simulink model "Main"  (R2020b)
settings: Solver=FixedStepAuto  StartTime=0.0  StopTime=60  FixedStep=0.01  RelTol=1e-3
settings Model: Creator=kaebi  LastModifiedBy=kaebi
settings OptimizationCC: DefaultParameterBehavior=Inlined  LocalBlockOutputs=off
settings RTWCC: Description=TwinCAT GRT Target  SystemTargetFile=TwinCatGrt.tlc  GenCodeOnly=on  TemplateMakefile=tcgrt_msbuild.tmf  TargetLang=C++
settings STFCustomTargetCC: TargetLangStandard=C++03 (ISO)  ConcurrentExecutionCompliant=off  CombineOutputUpdateFcns=on  CodeInterfacePackaging=Reusable function  GRTInterface=off  GenerateAllocFcn=on  SystemTargetFile=TwinCatGrt.tlc
settings GRTTargetCC: TargetLangStandard=C++03 (ISO)  ParMdlRefBuildCompliant=off  CompOptLevelCompliant=off  ConcurrentExecutionCompliant=off  MatFileLogging=off  CodeInterfacePackaging=Reusable function  GenerateAllocFcn=on  UseToolchainInfoCompliant=off  ExtModeMexFile=TcExtModeClient

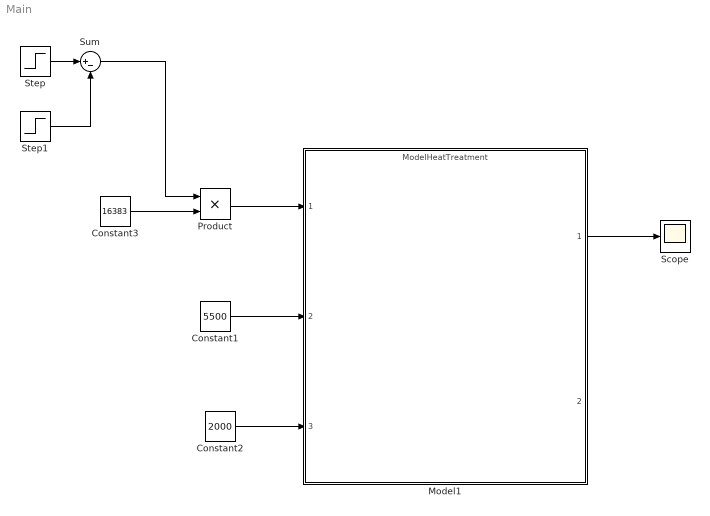
== system Main ==
  Constant1 : Constant  Value=5500  OutDataTypeStr=uint16
  Constant2 : Constant  Value=2000  OutDataTypeStr=uint16
  Constant3 : Constant  Value=16383  OutDataTypeStr=uint16
  Model1 : ModelReference  ModelNameDialog=ModelHeatTreatment.slx  SimulationMode=Normal  ModelReferenceVersion=1.35
  Product : Product  OutDataTypeStr=uint16
  Scope : Scope
  Step : Step  SampleTime=0
  Step1 : Step  Time=30  SampleTime=0
  Sum : Sum  Inputs=|+-
  wires:
  Model1/1 -> Scope/1
  Step/1 -> Sum/1
  Step1/1 -> Sum/2
  Product/1 -> Model1/1
  Constant3/1 -> Product/2
  Sum/1 -> Product/1
  Constant2/1 -> Model1/3
  Constant1/1 -> Model1/2
